simulink model "crazyflie"  (R2016b)
settings: Solver=FixedStepDiscrete  StartTime=0.0  StopTime=25  FixedStep=0.01  RelTol=1e-3
settings Model: PauseTimes=7  Creator=Zrean  LastModifiedBy=Zrean
settings OptimizationCC: DefaultParameterBehavior=Inlined  UseDivisionForNetSlopeComputation=on  UseFloatMulNetSlope=on  UseSpecifiedMinMax=on  InlineInvariantSignals=on  PassReuseOutputArgsAs=Individual arguments  ZeroExternalMemoryAtStartup=off  ZeroInternalMemoryAtStartup=off  NoFixptDivByZeroProtection=on  EfficientFloat2IntCast=on  LifeSpan=1
settings DebuggingCC: AlgebraicLoopMsg=error  ParameterTunabilityLossMsg=error
settings HardwareCC: ProdBitPerPointer=32  ProdBitPerSizeT=32  ProdBitPerPtrDiffT=32  ProdLargestAtomicInteger=Long  ProdLargestAtomicFloat=Double  ProdWordSize=32  ProdHWDeviceType=ARM Compatible->ARM Cortex
settings RTWCC: SystemTargetFile=ert.tlc  GenCodeOnly=on  TemplateMakefile=ert_default_tmf  Description=Embedded Coder  GenerateReport=on  Toolchain=GNU Tools for ARM Embedded Processors  BuildConfiguration=Faster Runs  IncludeHyperlinkInReport=on  LaunchReport=on  GenerateTraceInfo=on  GenerateTraceReport=on  GenerateTraceReportSl=on  GenerateTraceReportSf=on  GenerateTraceReportEml=on  GenerateCodeMetricsReport=on
settings CodeAppCC: ForceParamTrailComments=on  IgnoreCustomStorageClasses=off  OperatorAnnotations=on  SimulinkDataObjDesc=on  SFDataObjDesc=on  MATLABFcnDesc=on  CustomSymbolStrGlobalVar=rt$N$M  CustomSymbolStrType=$N$M  CustomSymbolStrFcn=$N$M$F  CustomSymbolStrMacro=$N$M  InsertBlockDesc=on  MATLABSourceComments=on
settings ERTTargetCC: TargetLangStandard=C99 (ISO)  CombineSignalStateStructs=on  SuppressErrorStatus=on  SupportAbsoluteTime=off  SupportNonFinite=off  SupportComplex=off  InlinedParameterPlacement=NonHierarchical  ERTCustomFileTemplate=crazyflie_wrapper.tlc  ERTFilePackagingFormat=CompactWithDataFile

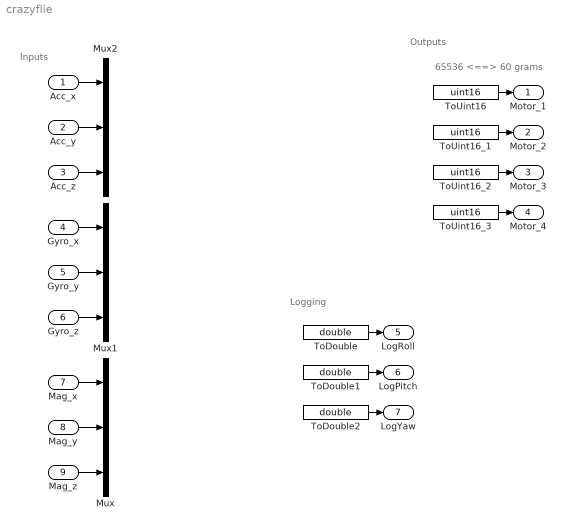
== system crazyflie ==
  note: 65536 <==> 60 grams
  note: Logging
  note: Outputs
  note: Inputs
  Acc_x : Inport  OutDataTypeStr=double  PortDimensions=1
  Acc_y : Inport  Port=2  OutDataTypeStr=double  PortDimensions=1
  Acc_z : Inport  Port=3  OutDataTypeStr=double  PortDimensions=1
  Gyro_x : Inport  Port=4  OutDataTypeStr=double  PortDimensions=1
  Gyro_y : Inport  Port=5  OutDataTypeStr=double  PortDimensions=1
  Gyro_z : Inport  Port=6  OutDataTypeStr=double  PortDimensions=1
  Mag_x : Inport  Port=7
  Mag_y : Inport  Port=8
  Mag_z : Inport  Port=9
  Mux : Mux  Inputs=3
  Mux1 : Mux  Inputs=3
  Mux2 : Mux  Inputs=3
  ToDouble : DataTypeConversion  OutDataTypeStr=double  SaturateOnIntegerOverflow=on
  ToDouble1 : DataTypeConversion  OutDataTypeStr=double  SaturateOnIntegerOverflow=on
  ToDouble2 : DataTypeConversion  OutDataTypeStr=double  SaturateOnIntegerOverflow=on
  ToUint16 : DataTypeConversion  OutDataTypeStr=uint16  SaturateOnIntegerOverflow=on
  ToUint16_1 : DataTypeConversion  OutDataTypeStr=uint16  SaturateOnIntegerOverflow=on
  ToUint16_2 : DataTypeConversion  OutDataTypeStr=uint16  SaturateOnIntegerOverflow=on
  ToUint16_3 : DataTypeConversion  OutDataTypeStr=uint16  SaturateOnIntegerOverflow=on
  Motor_1 : Outport  OutDataTypeStr=uint16  LockScale=on
  Motor_2 : Outport  Port=2  OutDataTypeStr=uint16  LockScale=on
  Motor_3 : Outport  Port=3  OutDataTypeStr=uint16  LockScale=on
  Motor_4 : Outport  Port=4  OutDataTypeStr=uint16  LockScale=on
  LogRoll : Outport  Port=5  OutDataTypeStr=double
  LogPitch : Outport  Port=6  OutDataTypeStr=double
  LogYaw : Outport  Port=7  OutDataTypeStr=double
  wires:
  Mag_y/1 -> Mux/2
  Mag_z/1 -> Mux/3
  Mag_x/1 -> Mux/1
  Gyro_x/1 -> Mux1/1
  Gyro_y/1 -> Mux1/2
  Gyro_z/1 -> Mux1/3
  Acc_x/1 -> Mux2/1
  Acc_z/1 -> Mux2/3
  Acc_y/1 -> Mux2/2
  ToUint16/1 -> Motor_1/1
  ToUint16_1/1 -> Motor_2/1
  ToUint16_2/1 -> Motor_3/1
  ToUint16_3/1 -> Motor_4/1
  ToDouble/1 -> LogRoll/1
  ToDouble1/1 -> LogPitch/1
  ToDouble2/1 -> LogYaw/1
